simulink model "GeneradorResiduos"  (R2022b)
settings: Solver=VariableStepAuto  StartTime=0.0  StopTime=10.0  RelTol=1e-3
values from neighbouring files (symbols this model uses):
  A = [-1 -2 ... (first row only)    [ABinvariantes11deJunio.m]    (also in Convertibility.m = [0 1 0  0 0; DivirsoresElementales.m = [1 0 -1; 0 1 0; 0 0 2]; Examen.m = [1 1;0 1]; Examen2.m = [0 0  0 0 0)
  B = [1 ... (first row only)    [ABinvariantes11deJunio.m]    (also in Convertibility.m = [0 0; Examen.m = [1;0]; Examen2.m = [1 0; Sestrella.m = [0;1;0])
  C = [1 0]    [Examen.m]    (also in Sestrella.m = [0 1 0; 0 0 1]; Westrella.m = [0 1 0; 0 0 1])
  Er = [-2 0]    [Westrella.m]
  Fr = -5    [Westrella.m]
  Gr = 1    [Westrella.m]
  H = D*inv((s*I-A+B*K))*B    [ABinvariantes11deJunio.m]    (also in Westrella.m = [1 -0;1 0])
  L = [0 ;0; 1]    [Sestrella.m]    (also in Westrella.m)
  L1 = [0;1;2]    [Westrella.m]
  Mr = [1;1]    [Westrella.m]
undefined symbols (not defined in the file or in its folder): sigbuilder_block
settings Model: Creator=raul  LastModifiedBy=raul

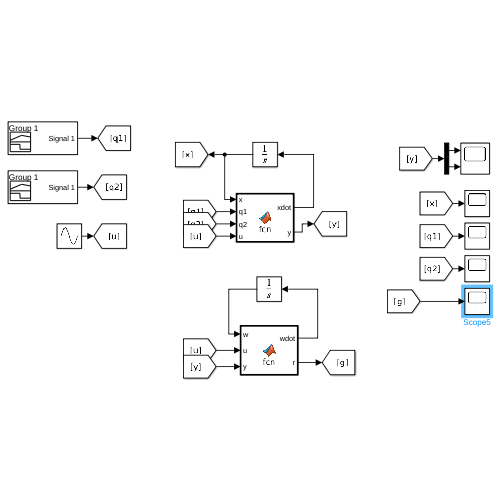
[thumbnail: Simulink's stored preview of the top-level diagram]
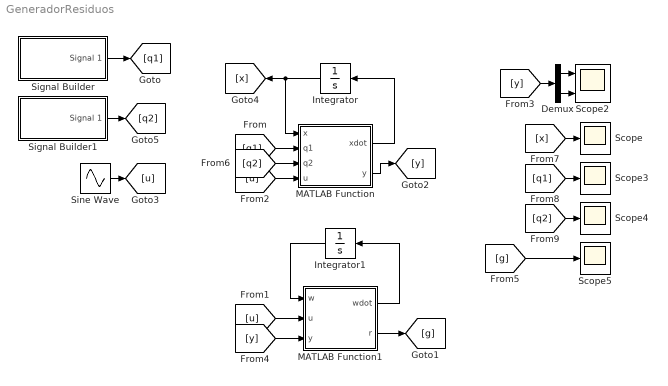
== system GeneradorResiduos ==
  Demux : Demux  Outputs=2
  Integrator : Integrator  InitialCondition=[0;0;0]
  Integrator1 : Integrator  InitialCondition=[0]
  MATLAB Function : MATLAB Function  TreatAsAtomicUnit=on
  MATLAB Function1 : MATLAB Function  TreatAsAtomicUnit=on
  Scope{,3..5} (4 alike) : Scope
  Scope2 : Scope  NumInputPorts=2
  Signal Builder : Subsystem  Tag=STV Subsys  LoadFcn=sigbuilder_block('load',[433.5 133.5 558 361.5 ]);  StartFcn=sigbuilder_block('start');  StopFcn=sigbuilder_block('stop');  ClipboardFcn=sigbuilder_block('clipboard');  mask(Sigbuilder block){tuvar=[0:10]}
      mask help: Simulink:masks:SigbuilderBlock_MD
      mask init:
      | if ~strcmp(get_param(bdroot(gcbh),'SimulationStatus'),'stopped') tuvar = sigbuilder_block('maskInit'); end
      settings: CopyFcn=sigbuilder_block('copy');  DeleteFcn=sigbuilder_block('delete');  ModelCloseFcn=sigbuilder_block('modelClose');  PreSaveFcn=sigbuilder_block('preSave');  PauseFcn=sigbuilder_block('pause');  ContinueFcn=sigbuilder_block('continue');  NameChangeFcn=sigbuilder_block('namechange');  OpenFcn=sigbuilder_block('open',[433.5 133.5 558 361.5 ]);  CloseFcn=sigbuilder_block('close');
      mask Display: plot(0, 0, 100, 100,[2, 2, 32, 32, 2], [68, 8, 8, 68, 68],[32, 2], [38, 38], [32, 19, 2],[53, 60, 44], [32, 17, 17, 2],[16, 16, 31, 31]);txt = getActiveGroup(gcbh);text(2, 100, txt,'verticalAlignment', 'top');
  Signal Builder1 : Subsystem  Tag=STV Subsys  LoadFcn=sigbuilder_block('load',[429.75 132.75 558 361.5 ]);  StartFcn=sigbuilder_block('start');  StopFcn=sigbuilder_block('stop');  ClipboardFcn=sigbuilder_block('clipboard');  mask(Sigbuilder block){tuvar=[0:10]}
      mask help: Simulink:masks:SigbuilderBlock_MD
      mask init:
      | if ~strcmp(get_param(bdroot(gcbh),'SimulationStatus'),'stopped') tuvar = sigbuilder_block('maskInit'); end
      settings: CopyFcn=sigbuilder_block('copy');  DeleteFcn=sigbuilder_block('delete');  ModelCloseFcn=sigbuilder_block('modelClose');  PreSaveFcn=sigbuilder_block('preSave');  PauseFcn=sigbuilder_block('pause');  ContinueFcn=sigbuilder_block('continue');  NameChangeFcn=sigbuilder_block('namechange');  OpenFcn=sigbuilder_block('open',[429.75 132.75 558 361.5 ]);  CloseFcn=sigbuilder_block('close');
      mask Display: plot(0, 0, 100, 100,[2, 2, 32, 32, 2], [68, 8, 8, 68, 68],[32, 2], [38, 38], [32, 19, 2],[53, 60, 44], [32, 17, 17, 2],[16, 16, 31, 31]);txt = getActiveGroup(gcbh);text(2, 100, txt,'verticalAlignment', 'top');
  Sine Wave : Sin  SampleTime=0
  wires:
  Signal Builder/1(Signal 1) -> [q1]
  MATLAB Function/1(xdot) -> Integrator/1
  MATLAB Function/2(y) -> [y]
  [q1] -> MATLAB Function/2(q1)
  [u] -> MATLAB Function/4(u)
  Integrator/1 -> [x], MATLAB Function/1(x)
  MATLAB Function1/1(wdot) -> Integrator1/1
  Integrator1/1 -> MATLAB Function1/1(w)
  [u] -> MATLAB Function1/2(u)
  [y] -> MATLAB Function1/3(y)
  MATLAB Function1/2(r) -> [g]
  [x] -> Scope/1
  Sine Wave/1 -> [u]
  Demux/1 -> Scope2/1
  Demux/2 -> Scope2/2
  [y] -> Demux/1
  [q2] -> MATLAB Function/3(q2)
  Signal Builder1/1(Signal 1) -> [q2]
  [q1] -> Scope3/1
  [q2] -> Scope4/1
  [g] -> Scope5/1

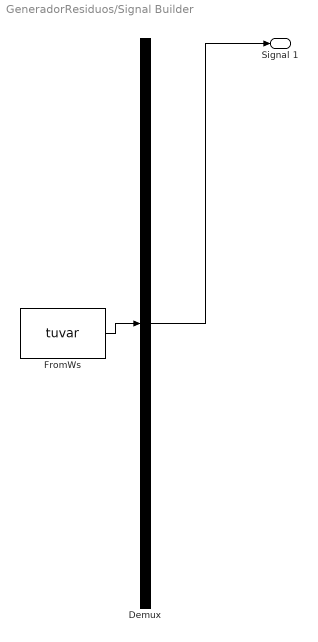
== system GeneradorResiduos/Signal Builder ==
  Demux : Demux  Tag=STV Demux  Outputs=1
      settings: DisplayOption=none
  FromWs : FromWorkspace  Tag=STV FromWs  VariableName=tuvar
      SigBuilderData=|
      | common.afterFinalStr = 'Extrapolate'
      | common.sampleTime = 0
      | dataSet.timeRange = [0 10]
      | dataSet.name = 'Group 1'
      | sbobj.Groups.Name = 'Group 1'
      | sbobj.Groups.Signals.Name = 'Signal 1'
      | sbobj.Groups.Signals.XData = [0 4 4 6 6 10]
      | sbobj.Groups.Signals.YData = [0 0 1 1 0 0]
  Signal 1 : Outport  Tag=STV Outport
  wires:
  Demux/1 -> Signal 1/1
  FromWs/1 -> Demux/1

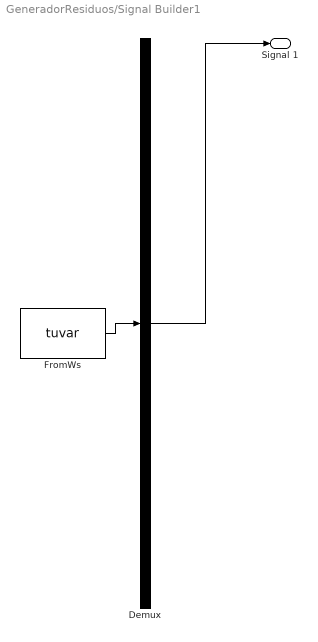
== system GeneradorResiduos/Signal Builder1 ==
  Demux : Demux  Tag=STV Demux  Outputs=1
      settings: DisplayOption=none
  FromWs : FromWorkspace  Tag=STV FromWs  VariableName=tuvar
      SigBuilderData=|
      | common.afterFinalStr = 'Extrapolate'
      | common.sampleTime = 0
      | dataSet.timeRange = [0 10]
      | dataSet.name = 'Group 1'
      | sbobj.Groups.Name = 'Group 1'
      | sbobj.Groups.Signals.Name = 'Signal 1'
      | sbobj.Groups.Signals.XData = [0 2.02 2.02 3.02 3.02 10]
      | sbobj.Groups.Signals.YData = [0 0 1 1 0 0]
  Signal 1 : Outport  Tag=STV Outport
  wires:
  Demux/1 -> Signal 1/1
  FromWs/1 -> Demux/1

== matlab function GeneradorResiduos/MATLAB Function1 ==
  data: wdot output; w input; u input; y input; r output; Fr parameter; Mr parameter; Gr parameter; Er parameter; H parameter
function [wdot,r] = fcn(w,u,y,Fr, Mr, Gr, Er,H)

wdot=Fr*w+Gr*u-Er*y;
r=Mr*w-H*y;

== matlab function GeneradorResiduos/MATLAB Function ==
  data: x input; xdot output; q1 input; q2 input; u input; y output; A parameter; B parameter; C parameter; L parameter; L1 parameter
function [xdot,y] = fcn(x,q1,q2,u,A, B, C, L, L1)

xdot=A*x+B*u+L1*q1+L*q2;
y=C*x;
